simulink model "PO10045"  (Simulink 7.5)
settings: Solver=ode23tb  StartTime=0.0  StopTime=0.16  MaxStep=5e-6  RelTol=1e-3
undefined symbols (not defined in the file or in its folder): sigbuilder_block
libraries: powerlib x11, simulink x1
settings Model: Creator=Administrator  LastModifiedBy=Administrator

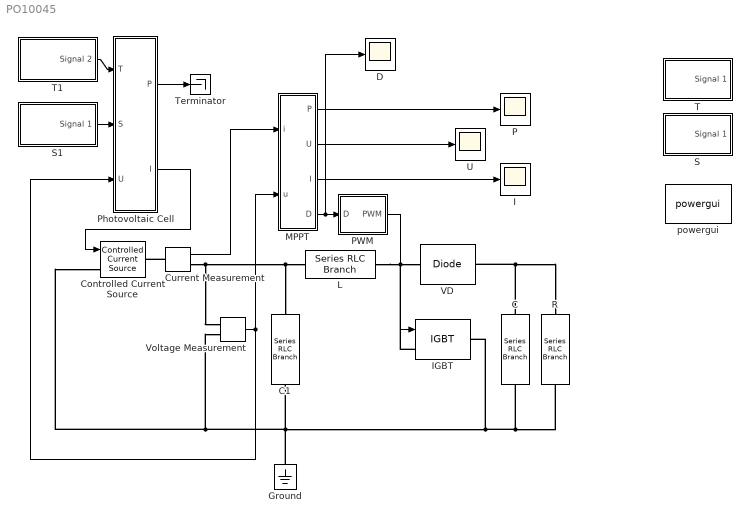
== system PO10045 ==
  C : powerlib/Elements/Series RLC Branch  DialogController=POWERSYS.PowerSysDialog  PhysicalDomain=powersysdomain  SubClassName=unknown  LeftPortType=p1  RightPortType=p1  LConnTagsString=__new0  RConnTagsString=__new0  BranchType=C  Resistance=0  Inductance=0  SetiL0=off  InitialCurrent=0  Capacitance=300e-6  Setx0=on  InitialVoltage=0  Measurements=None
  C1 : powerlib/Elements/Series RLC Branch  DialogController=POWERSYS.PowerSysDialog  PhysicalDomain=powersysdomain  SubClassName=unknown  LeftPortType=p1  RightPortType=p1  LConnTagsString=__new0  RConnTagsString=__new0  BranchType=C  Resistance=0  Inductance=0  SetiL0=off  InitialCurrent=0  Capacitance=300e-6  Setx0=off  InitialVoltage=0  Measurements=None
  Controlled Current Source : powerlib/Electrical Sources/Controlled Current Source  DialogController=POWERSYS.PowerSysDialog  SystemSampleTime=-1  Initialize=on  Source_Type=DC  Amplitude=0  Phase=0  Frequency=0  Measurements=None
  Current Measurement : powerlib/Measurements/Current Measurement  DialogController=POWERSYS.PowerSysDialog  SystemSampleTime=-1  PhasorSimulation=off  OutputType=Complex  PSBequivalent=0
  D : Scope
      settings: TimeRange=0.008767576509512001  YMin=5.469352014010505  YMax=10.45008756567425  SaveName=U1
  Ground : powerlib/Elements/Ground  DialogController=POWERSYS.PowerSysDialog  PhysicalDomain=powersysdomain  SubClassName=unknown  LeftPortType=p1  RightPortType=p1  LConnTagsString=a
  I : Scope
      settings: YMin=0.795  YMax=0.805  SaveName=I
  IGBT : powerlib/Power Electronics/IGBT  DialogController=POWERSYS.PowerSysDialog  SystemSampleTime=-1  Ron=0.00000001  Lon=0  Vf=1  Tf=1e-6  Tt=2e-6  IC=0  Rs=1e5  Cs=inf  Measurements=off
  L : powerlib/Elements/Series RLC Branch  DialogController=POWERSYS.PowerSysDialog  PhysicalDomain=powersysdomain  SubClassName=unknown  LeftPortType=p1  RightPortType=p1  LConnTagsString=__new0  RConnTagsString=__new0  BranchType=L  Resistance=0  Inductance=200e-6  SetiL0=off  InitialCurrent=1  Capacitance=inf  Setx0=off  InitialVoltage=0  Measurements=None
  "MPPT " : Subsystem
  P : Scope
      settings: TimeRange=0.008767576509512001  YMin=5.469352014010505  YMax=10.45008756567425  SaveName=U
  PWM : Subsystem
  Photovoltaic Cell : Subsystem  mask(Photovoltaic Cell){a=0.00398, b=0.0821, Rs=0.5, Isc=1, Uoc=21.7, Im=0.91, Um=17.6, Sref=1000, Tref=25}
  R : powerlib/Elements/Series RLC Branch  DialogController=POWERSYS.PowerSysDialog  PhysicalDomain=powersysdomain  SubClassName=unknown  LeftPortType=p1  RightPortType=p1  LConnTagsString=__new0  RConnTagsString=__new0  BranchType=R  Resistance=30  Inductance=100e-6  SetiL0=off  InitialCurrent=0  Capacitance=inf  Setx0=off  InitialVoltage=0  Measurements=None
  S : Subsystem  Tag=STV Subsys  LoadFcn=sigbuilder_block('load');  StartFcn=sigbuilder_block('start');  StopFcn=sigbuilder_block('stop');  ClipboardFcn=sigbuilder_block('clipboard');  mask(Sigbuilder block){}
      mask help: Sigbuilder GUI
      mask init:
      | if ~strcmp(get_param(bdroot(gcbh),'SimulationStatus'),'stopped') tuvar = sigbuilder_block('maskInit'); end
      settings: CopyFcn=sigbuilder_block('copy');  DeleteFcn=sigbuilder_block('delete');  ModelCloseFcn=sigbuilder_block('modelClose');  PreSaveFcn=sigbuilder_block('preSave');  NameChangeFcn=sigbuilder_block('namechange');  OpenFcn=sigbuilder_block('open',[120.414 93.1034 518.897 339.517 ]);  CloseFcn=sigbuilder_block('close');
      mask Display: plot(0,0,100,100,[10,10,40,40,10],[80,20,20,80,80],[40,10],[50,50], [40,27,10],[65,72,56],[40,25,25,10],[28,28,43,43]);
  S1 : Subsystem  Tag=STV Subsys  LoadFcn=sigbuilder_block('load');  StartFcn=sigbuilder_block('start');  StopFcn=sigbuilder_block('stop');  ClipboardFcn=sigbuilder_block('clipboard');  mask(Sigbuilder block){}
      mask help: Sigbuilder GUI
      mask init:
      | if ~strcmp(get_param(bdroot(gcbh),'SimulationStatus'),'stopped') tuvar = sigbuilder_block('maskInit'); end
      settings: CopyFcn=sigbuilder_block('copy');  DeleteFcn=sigbuilder_block('delete');  ModelCloseFcn=sigbuilder_block('modelClose');  PreSaveFcn=sigbuilder_block('preSave');  NameChangeFcn=sigbuilder_block('namechange');  OpenFcn=sigbuilder_block('open',[50.2759 41.5862 518.897 397.241 ]);  CloseFcn=sigbuilder_block('close');
      mask Display: plot(0,0,100,100,[10,10,40,40,10],[80,20,20,80,80],[40,10],[50,50], [40,27,10],[65,72,56],[40,25,25,10],[28,28,43,43]);
  T : Subsystem  Tag=STV Subsys  LoadFcn=sigbuilder_block('load');  StartFcn=sigbuilder_block('start');  StopFcn=sigbuilder_block('stop');  ClipboardFcn=sigbuilder_block('clipboard');  mask(Sigbuilder block){}
      mask help: Sigbuilder GUI
      mask init:
      | if ~strcmp(get_param(bdroot(gcbh),'SimulationStatus'),'stopped') tuvar = sigbuilder_block('maskInit'); end
      settings: CopyFcn=sigbuilder_block('copy');  DeleteFcn=sigbuilder_block('delete');  ModelCloseFcn=sigbuilder_block('modelClose');  PreSaveFcn=sigbuilder_block('preSave');  NameChangeFcn=sigbuilder_block('namechange');  OpenFcn=sigbuilder_block('open',[142.759 39.1034 519.517 399.724 ]);  CloseFcn=sigbuilder_block('close');
      mask Display: plot(0,0,100,100,[10,10,40,40,10],[80,20,20,80,80],[40,10],[50,50], [40,27,10],[65,72,56],[40,25,25,10],[28,28,43,43]);
  T1 : Subsystem  Tag=STV Subsys  LoadFcn=sigbuilder_block('load');  StartFcn=sigbuilder_block('start');  StopFcn=sigbuilder_block('stop');  ClipboardFcn=sigbuilder_block('clipboard');  mask(Sigbuilder block){}
      mask help: Sigbuilder GUI
      mask init:
      | if ~strcmp(get_param(bdroot(gcbh),'SimulationStatus'),'stopped') tuvar = sigbuilder_block('maskInit'); end
      settings: CopyFcn=sigbuilder_block('copy');  DeleteFcn=sigbuilder_block('delete');  ModelCloseFcn=sigbuilder_block('modelClose');  PreSaveFcn=sigbuilder_block('preSave');  NameChangeFcn=sigbuilder_block('namechange');  OpenFcn=sigbuilder_block('open',[142.759 39.1034 519.517 399.724 ]);  CloseFcn=sigbuilder_block('close');
      mask Display: plot(0,0,100,100,[10,10,40,40,10],[80,20,20,80,80],[40,10],[50,50], [40,27,10],[65,72,56],[40,25,25,10],[28,28,43,43]);
  Terminator : Terminator
  U : Scope
      settings: YMin=3.02619  YMax=3.34473  SaveName=I1
  VD : powerlib/Power Electronics/Diode  DialogController=POWERSYS.PowerSysDialog  SystemSampleTime=-1  Ron=0.00000001  Lon=0  Vf=0.7  IC=0  UseSnubber=off  Rs=500  Cs=250e-9  Measurements=off
  Voltage Measurement : powerlib/Measurements/Voltage Measurement  DialogController=POWERSYS.PowerSysDialog  SystemSampleTime=-1  PhasorSimulation=off  OutputType=Complex  PSBequivalent=0
  powergui : powerlib/powergui  Priority=1  SystemSampleTime=-1  SimulationMode=Discrete  SampleTime=50e-8  frequency=60  SPID=off  DisableSnubberDevices=off  DisableRonSwitches=off  DisableVfSwitches=off  SwTol=0  Interpol=off  frequencyindice=0  echomessages=off  HookPort=off  DisplayEquations=off  FunctionMessages=off  EnableUseOfTLC=off  x0status=blocks  RestoreLinks=warning  ResistiveCurrentMeasurement=off  Ylog=off  Xlog=on  ShowGrid=off  save=off  variable=ZData  ZoomFFT=off  StartTime=0.0  cycles=1  DisplayStyle=1  FreqAxis=off  MaxFrequency=1000  frequencyindicesteady=1  display=off  methode=off
  wires:
  Photovoltaic Cell/2(I) -> Controlled Current Source/1
  Voltage Measurement/1 -> "MPPT "/2(u), Photovoltaic Cell/3(U)
  Photovoltaic Cell/1(P) -> Terminator/1
  T1/1(Signal 2) -> Photovoltaic Cell/1(T)
  S1/1(Signal 1) -> Photovoltaic Cell/2(S)
  Current Measurement/1 -> "MPPT "/1(i)
  "MPPT "/4(D) -> PWM/1(D), D/1
  "MPPT "/1(P) -> P/1
  "MPPT "/2(U) -> U/1
  "MPPT "/3(I) -> I/1
  PWM/1(PWM) -> IGBT/1
  connections:
  L/RConn1 -- IGBT/LConn1 -- VD/LConn1
  VD/RConn1 -- R/LConn1 -- C/LConn1
  Voltage Measurement/LConn1 -- Current Measurement/RConn1 -- C1/LConn1 -- L/LConn1
  C1/RConn1 -- Controlled Current Source/LConn1 -- Voltage Measurement/LConn2 -- Ground/LConn1 -- C/RConn1 -- R/RConn1 -- IGBT/RConn1
  Current Measurement/LConn1 -- Controlled Current Source/RConn1

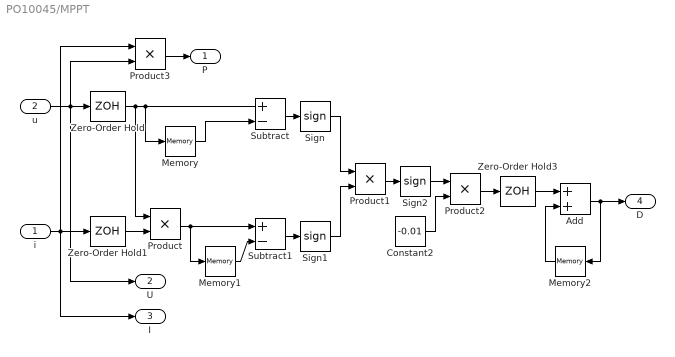
== system PO10045/MPPT  ==
  i : Inport  OutDataType=sfix(16)  OutScaling=2^0
  u : Inport  Port=2  OutDataType=sfix(16)  OutScaling=2^0
  Add : Sum  OutDataType=sfix(16)  OutScaling=2^-10
  Constant2 : Constant  Value=-0.01  OutDataType=sfix(16)  OutScaling=2^0
  Memory : Memory  InheritSampleTime=on
  Memory1 : Memory  InheritSampleTime=on
  Memory2 : Memory  X0=1  InheritSampleTime=on
  Product{,1..3} (4 alike) : Product  OutDataType=sfix(16)  OutScaling=2^0  RndMeth=Zero
  Sign : Signum
  Sign1 : Signum
  Sign2 : Signum
  Subtract : Sum  Inputs=+-  OutDataType=sfix(16)  OutScaling=2^-10
  Subtract1 : Sum  Inputs=+-  OutDataType=sfix(16)  OutScaling=2^-10
  Zero-Order Hold : ZeroOrderHold  SampleTime=0.0005
  Zero-Order Hold1 : ZeroOrderHold  SampleTime=0.0005
  Zero-Order Hold3 : ZeroOrderHold  SampleTime=0.0005
  P : Outport  OutDataType=sfix(16)  OutScaling=2^0
  U : Outport  Port=2  OutDataType=sfix(16)  OutScaling=2^0
  I : Outport  Port=3  OutDataType=sfix(16)  OutScaling=2^0
  D : Outport  Port=4  OutDataType=sfix(16)  OutScaling=2^0
  wires:
  u/1 -> Zero-Order Hold/1, Product3/2, U/1
  i/1 -> Zero-Order Hold1/1, Product3/1, I/1
  Zero-Order Hold/1 -> Product/1, Subtract/1, Memory/1
  Memory/1 -> Subtract/2
  Zero-Order Hold1/1 -> Product/2
  Product/1 -> Subtract1/1, Memory1/1
  Memory1/1 -> Subtract1/2
  Subtract/1 -> Sign/1
  Subtract1/1 -> Sign1/1
  Sign/1 -> Product1/1
  Sign1/1 -> Product1/2
  Product1/1 -> Sign2/1
  Sign2/1 -> Product2/1
  Add/1 -> Memory2/1, D/1
  Memory2/1 -> Add/2
  Constant2/1 -> Product2/2
  Product3/1 -> P/1
  Product2/1 -> Zero-Order Hold3/1
  Zero-Order Hold3/1 -> Add/1

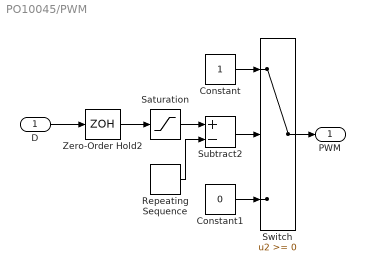
== system PO10045/PWM ==
  D : Inport  OutDataType=sfix(16)  OutScaling=2^0
  Constant : Constant  OutDataType=sfix(16)  OutScaling=2^0
  Constant1 : Constant  Value=0  OutDataType=sfix(16)  OutScaling=2^0
  Repeating Sequence : simulink/Sources/Repeating Sequence  SystemSampleTime=-1  rep_seq_t=[0 0.0001]  rep_seq_y=[0 1]
  Saturation : Saturate  UpperLimit=1  LowerLimit=0
  Subtract2 : Sum  Inputs=+-  OutDataType=sfix(16)  OutScaling=2^-10
  Switch : Switch
  Zero-Order Hold2 : ZeroOrderHold  SampleTime=0.0005
  PWM : Outport  OutDataType=sfix(16)  OutScaling=2^0
  wires:
  Zero-Order Hold2/1 -> Saturation/1
  Switch/1 -> PWM/1
  Constant1/1 -> Switch/3
  Constant/1 -> Switch/1
  Subtract2/1 -> Switch/2
  Repeating Sequence/1 -> Subtract2/2
  Saturation/1 -> Subtract2/1
  D/1 -> Zero-Order Hold2/1

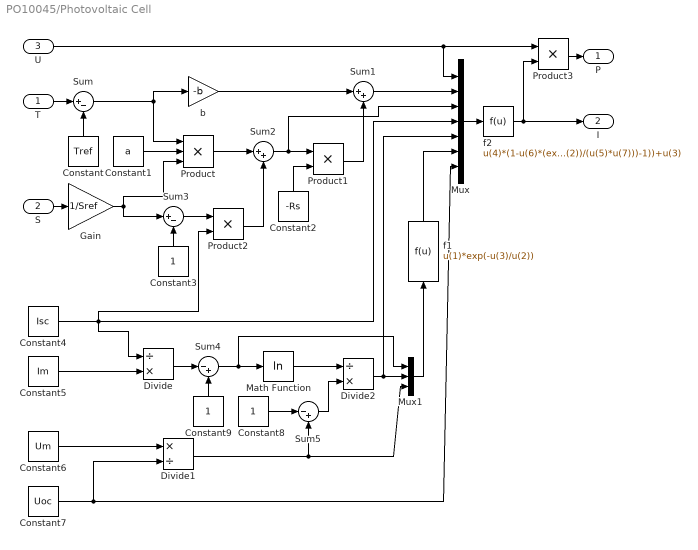
== system PO10045/Photovoltaic Cell ==
  T : Inport  OutDataType=sfix(16)  OutScaling=2^0
  S : Inport  Port=2  OutDataType=sfix(16)  OutScaling=2^0
  U : Inport  Port=3  OutDataType=sfix(16)  OutScaling=2^0
  Constant : Constant  Value=Tref  OutDataType=sfix(16)  OutScaling=2^0
  Constant1 : Constant  Value=a  OutDataType=sfix(16)  OutScaling=2^0
  Constant2 : Constant  Value=-Rs  OutDataType=sfix(16)  OutScaling=2^0
  Constant3 : Constant  OutDataType=sfix(16)  OutScaling=2^0
  Constant4 : Constant  Value=Isc  OutDataType=sfix(16)  OutScaling=2^0
  Constant5 : Constant  Value=Im  OutDataType=sfix(16)  OutScaling=2^0
  Constant6 : Constant  Value=Um  OutDataType=sfix(16)  OutScaling=2^0
  Constant7 : Constant  Value=Uoc  OutDataType=sfix(16)  OutScaling=2^0
  Constant8 : Constant  OutDataType=sfix(16)  OutScaling=2^0
  Constant9 : Constant  OutDataType=sfix(16)  OutScaling=2^0
  Divide : Product  Inputs=/*  OutDataType=sfix(16)  OutScaling=2^-10
  Divide1 : Product  Inputs=*/  OutDataType=sfix(16)  OutScaling=2^-10
  Divide2 : Product  Inputs=/*  OutDataType=sfix(16)  OutScaling=2^-10
  Gain : Gain  Gain=1/Sref  ParameterDataType=sfix(16)  ParameterScaling=2^0  OutDataType=sfix(16)  OutScaling=2^0
  Math Function : Math  Operator=log  OutDataType=sfix(16)  OutScaling=2^0  SaturateOnIntegerOverflow=on
  Mux : Mux  Inputs=7
  Mux1 : Mux  Inputs=3
  Product : Product  Inputs=3  OutDataType=sfix(16)  OutScaling=2^0  RndMeth=Zero
  Product1 : Product  OutDataType=sfix(16)  OutScaling=2^0  RndMeth=Zero
  Product2 : Product  OutDataType=sfix(16)  OutScaling=2^0  RndMeth=Zero
  Product3 : Product  OutDataType=sfix(16)  OutScaling=2^0  RndMeth=Zero
  Sum : Sum  Inputs=|+-  OutDataType=sfix(16)  OutScaling=2^0
  Sum1 : Sum  Inputs=|++  OutDataType=sfix(16)  OutScaling=2^0
  Sum2 : Sum  Inputs=|++  OutDataType=sfix(16)  OutScaling=2^0
  Sum3 : Sum  Inputs=|+-  OutDataType=sfix(16)  OutScaling=2^0
  Sum4 : Sum  Inputs=|-+  OutDataType=sfix(16)  OutScaling=2^0
  Sum5 : Sum  Inputs=|-+  OutDataType=sfix(16)  OutScaling=2^0
  b : Gain  Gain=-b  ParameterDataType=sfix(16)  ParameterScaling=2^0  OutDataType=sfix(16)  OutScaling=2^0
  f1 : Fcn  Expr=u(1)*exp(-u(3)/u(2))
  f2 : Fcn  Expr=u(4)*(1-u(6)*(exp((u(1)-u(2))/(u(5)*u(7)))-1))+u(3)
  P : Outport  OutDataType=sfix(16)  OutScaling=2^0
  I : Outport  Port=2  OutDataType=sfix(16)  OutScaling=2^0
  wires:
  T/1 -> Sum/1
  Sum/1 -> Product/1, b/1
  b/1 -> Sum1/1
  Constant/1 -> Sum/2
  S/1 -> Gain/1
  Gain/1 -> Product/3, Sum3/1
  Constant1/1 -> Product/2
  Product/1 -> Sum2/1
  Sum2/1 -> Product1/1, Mux/3
  Constant2/1 -> Product1/2
  Sum3/1 -> Product2/1
  Product2/1 -> Sum2/2
  Constant3/1 -> Sum3/2
  Product1/1 -> Sum1/2
  Constant4/1 -> Product2/2, Mux/4, Divide/1
  Sum1/1 -> Mux/2
  U/1 -> Mux/1, Product3/1
  Divide/1 -> Sum4/1
  Constant9/1 -> Sum4/2
  Constant5/1 -> Divide/2
  Constant7/1 -> Divide1/2, Mux/7
  Constant6/1 -> Divide1/1
  Sum4/1 -> Math Function/1, Mux1/1
  Divide1/1 -> Sum5/2, Mux1/3
  Constant8/1 -> Sum5/1
  Sum5/1 -> Divide2/2
  Math Function/1 -> Divide2/1
  Divide2/1 -> Mux1/2, Mux/5
  Mux1/1 -> f1/1
  f1/1 -> Mux/6
  Mux/1 -> f2/1
  Product3/1 -> P/1
  f2/1 -> I/1, Product3/2

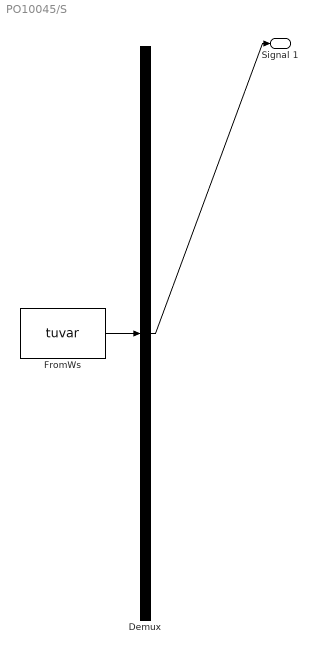
== system PO10045/S ==
  Demux : Demux  Tag=STV Demux  Outputs=1
  FromWs : FromWorkspace  Tag=STV FromWs  VariableName=tuvar  SampleTime=0  SigBuilderData=DataTag0  VnvData=DataTag1
      SigBuilderData=|
      | dataSet.timeRange = [0 0.16]
      | dataSet.name = 'Group 1'
      | sbobj.Groups.Name = 'Group 1'
      | sbobj.Groups.Signals.Name = 'Signal 1'
      | sbobj.Groups.Signals.XData = [0 0.1 0.1 0.16]
      | sbobj.Groups.Signals.YData = [1000 1000 800 800]
  Signal 1 : Outport  Tag=STV Outport  OutDataType=sfix(16)  OutScaling=2^0
  wires:
  Demux/1 -> Signal 1/1
  FromWs/1 -> Demux/1

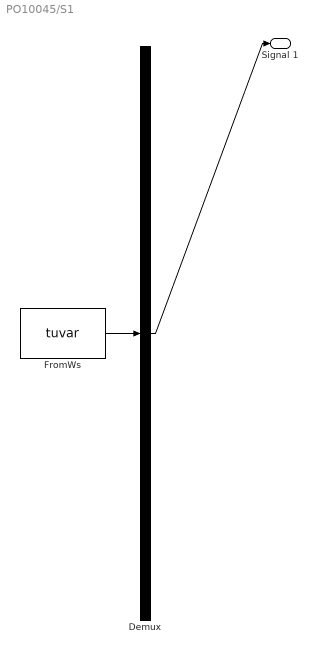
== system PO10045/S1 ==
  Demux : Demux  Tag=STV Demux  Outputs=1
  FromWs : FromWorkspace  Tag=STV FromWs  VariableName=tuvar  SampleTime=0  SigBuilderData=DataTag2  VnvData=DataTag3
      SigBuilderData=|
      | dataSet.timeRange = [0 0.16]
      | dataSet.name = 'Group 1'
      | sbobj.Groups.Name = 'Group 1'
      | sbobj.Groups.Signals.Name = 'Signal 1'
      | sbobj.Groups.Signals.XData = [0 0.05 0.16]
      | sbobj.Groups.Signals.YData = [1000 1000 1000]
  Signal 1 : Outport  Tag=STV Outport  OutDataType=sfix(16)  OutScaling=2^0
  wires:
  Demux/1 -> Signal 1/1
  FromWs/1 -> Demux/1

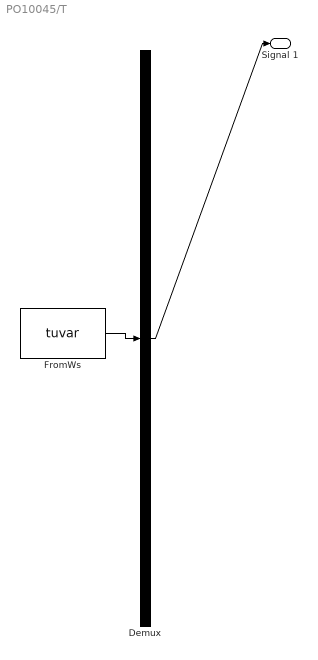
== system PO10045/T ==
  Demux : Demux  Tag=STV Demux  Outputs=1
  FromWs : FromWorkspace  Tag=STV FromWs  VariableName=tuvar  SampleTime=0  SigBuilderData=DataTag4  VnvData=DataTag5
      SigBuilderData=|
      | dataSet.timeRange = [0 0.16]
      | dataSet.name = 'Group 1'
      | sbobj.Groups.Name = 'Group 1'
      | sbobj.Groups.Signals.Name = 'Signal 1'
      | sbobj.Groups.Signals.XData = [0 0.16]
      | sbobj.Groups.Signals.YData = [25 25]
  Signal 1 : Outport  Tag=STV Outport  OutDataType=sfix(16)  OutScaling=2^0
  wires:
  FromWs/1 -> Demux/1
  Demux/1 -> Signal 1/1

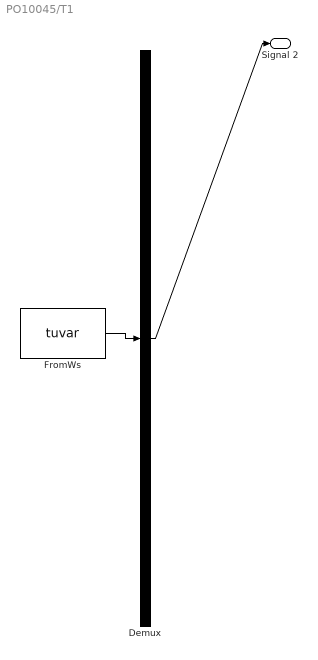
== system PO10045/T1 ==
  Demux : Demux  Tag=STV Demux  Outputs=1
  FromWs : FromWorkspace  Tag=STV FromWs  VariableName=tuvar  SampleTime=0  SigBuilderData=DataTag6  VnvData=DataTag7
      SigBuilderData=|
      | dataSet.timeRange = [0 0.16]
      | dataSet.name = 'Group 1'
      | sbobj.Groups.Name = 'Group 1'
      | sbobj.Groups.Signals.Name = 'Signal 2'
      | sbobj.Groups.Signals.XData = [0 0.1 0.1 0.16]
      | sbobj.Groups.Signals.YData = [25 25 45 45]
  Signal 2 : Outport  Tag=STV Outport  OutDataType=sfix(16)  OutScaling=2^0
  wires:
  FromWs/1 -> Demux/1
  Demux/1 -> Signal 2/1
